simulink model "Laplace"  (R2020a)
settings: Solver=VariableStepAuto  StartTime=0.0  StopTime=10.0  RelTol=1e-3
settings Model: Creator=Mohammad  LastModifiedBy=Mohammad

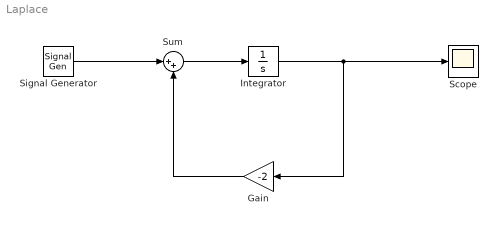
== system Laplace ==
  Gain : Gain  Gain=-2
  Integrator : Integrator
  Scope : Scope
  Signal Generator : SignalGenerator  WaveForm=square  Units=rad/sec
  Sum : Sum  Inputs=|++
  wires:
  Integrator/1 -> Gain/1, Scope/1
  Sum/1 -> Integrator/1
  Gain/1 -> Sum/2
  Signal Generator/1 -> Sum/1
